simulink library "Centralized_I_Lib_Controller"  (R2024b)
settings: Solver=VariableStepAuto  StartTime=0.0  StopTime=10.0  RelTol=1e-3
(part 1 of 7)
settings Model: Creator=pepev  LastModifiedBy=pepev

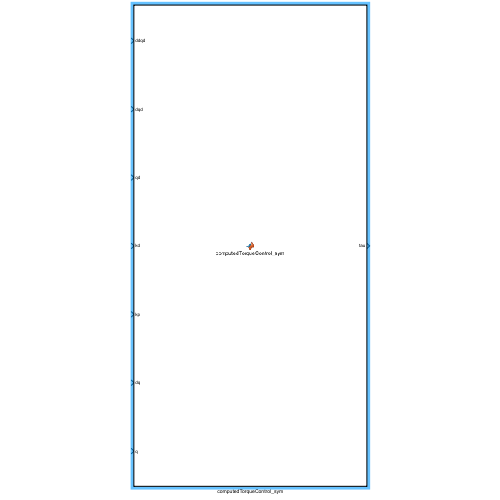
[thumbnail: Simulink's stored preview of the top-level diagram]
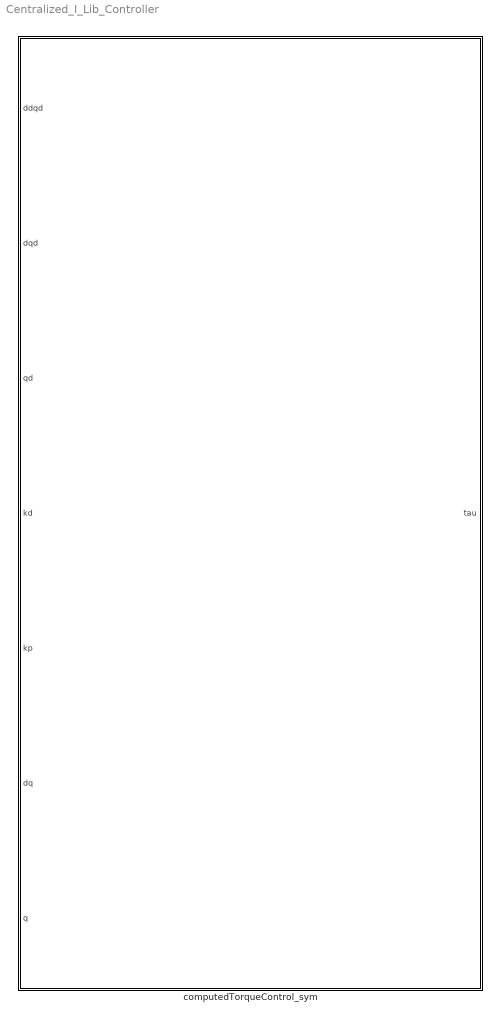
== system Centralized_I_Lib_Controller ==
  computedTorqueControl_sym : MATLAB Function  TreatAsAtomicUnit=on
